simulink model "Test_LQG_non_linear"  (R2022b)
settings: Solver=VariableStepAuto  StartTime=0.0  StopTime=100.0  RelTol=1e-3
values from neighbouring files (symbols this model uses):
  a = Mv+mp+2*ma+2*IAy/(ra^2)    (= 19.1666666667)    [function_f.m]
  b = 1/2*(Mv*l^2+mp*L^2+2*ma*d^2+IGz+IPz+2*IAz+2*IAy*(d/ra)^2)    (= 3.3525)    [function_f.m]
  IPy = 0.15    [function_f.m]
  IPz = 0.23    [function_f.m]
  J = get_linearization()    [DK_iteration.m]    (also in LQG.m; LQG_integrator.m; LQG_with_integrator.m; mu_analysis.m = get_linearization_lqg())
  Kr = lqr(J.A,J.B,Q,R)    [LQG.m]    (also in LQG_integrator.m = lqr(A,B,Q,R); LQG_with_integrator.m = lqr(A,B,Q,R))
  L = 1    [function_f.m]
  rp = 0.3    [function_f.m]
undefined symbols (not defined in the file or in its folder): Ke, std_dev_dx, std_dev_dy, std_dev_phi_dot, std_dev_psi, X_start
libraries: simulink x2
settings Model: Creator=alexi  LastModifiedBy=alexi

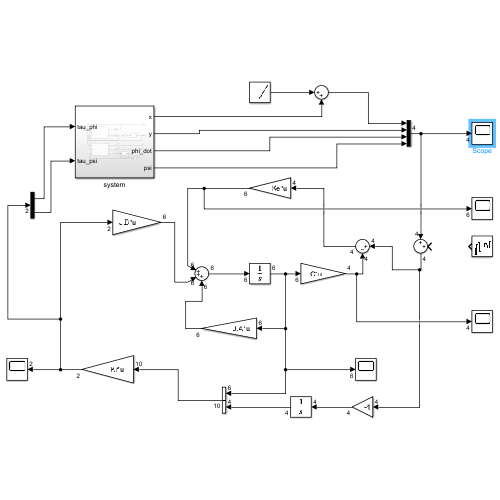
[thumbnail: Simulink's stored preview of the top-level diagram]
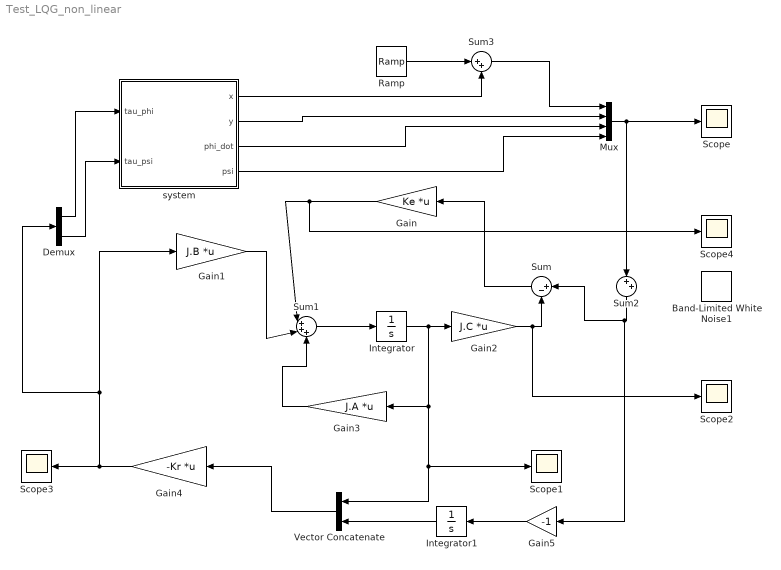
== system Test_LQG_non_linear ==
  Band-Limited White Noise1 : simulink/Sources/Band-Limited White Noise  Cov=[std_dev_dx; std_dev_dy; std_dev_phi_dot; std_dev_psi]  Ts=0.1  seed=[23341]
  Demux : Demux  Outputs=2
  Gain : Gain  Gain=Ke  Multiplication=Matrix(K*u)
  Gain1 : Gain  Gain=J.B  Multiplication=Matrix(K*u)
  Gain2 : Gain  Gain=J.C  Multiplication=Matrix(K*u)
  Gain3 : Gain  Gain=J.A  Multiplication=Matrix(K*u)
  Gain4 : Gain  Gain=-Kr  Multiplication=Matrix(K*u)
  Gain5 : Gain  Gain=-1
  Integrator : Integrator
  Integrator1 : Integrator
  Mux : Mux
  Ramp : simulink/Sources/Ramp  slope=1  start=0  InitialOutput=0
  Scope{,1..4} (5 alike) : Scope
  Sum : Sum  Inputs=|+-
  Sum1 : Sum  Inputs=|+++
  Sum2 : Sum  Inputs=|++
  Sum3 : Sum  Inputs=|++
  Vector Concatenate : Concatenate
  system : Subsystem
  wires:
  Sum1/1 -> Integrator/1
  Gain1/1 -> Sum1/2
  Sum/1 -> Gain/1
  Gain3/1 -> Sum1/3
  Sum2/1 -> Gain5/1, Sum/1
  Integrator/1 -> Vector Concatenate/1, Scope1/1, Gain3/1, Gain2/1
  Gain/1 -> Scope4/1, Sum1/1
  Gain2/1 -> Scope2/1, Sum/2
  Gain4/1 -> Demux/1, Gain1/1, Scope3/1
  Gain5/1 -> Integrator1/1
  Vector Concatenate/1 -> Gain4/1
  Integrator1/1 -> Vector Concatenate/2
  Mux/1 -> Scope/1, Sum2/1
  system/1(x) -> Sum3/2
  Sum3/1 -> Mux/1
  Ramp/1 -> Sum3/1
  system/2(y) -> Mux/2
  system/3(phi_dot) -> Mux/3
  system/4(psi) -> Mux/4
  Demux/1 -> system/1(tau_phi)
  Demux/2 -> system/2(tau_psi)

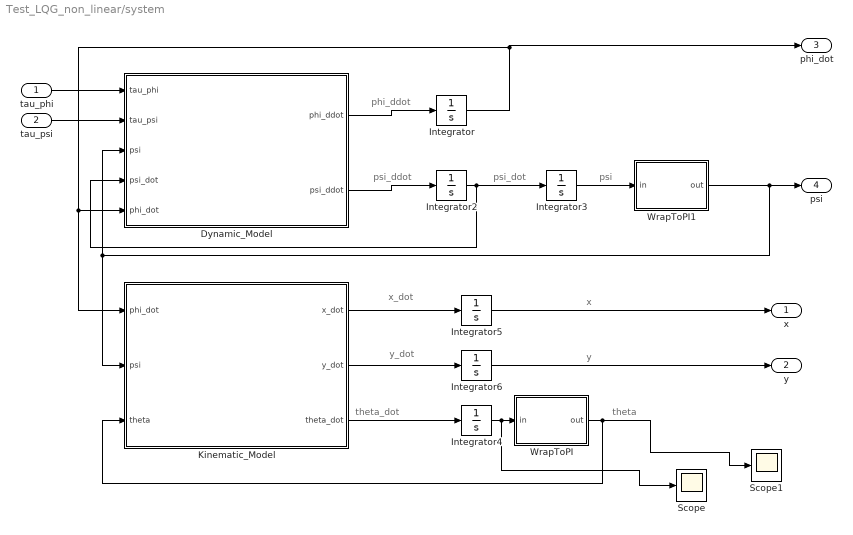
== system Test_LQG_non_linear/system ==
  note: theta_dot
  note: psi_dot
  note: psi_ddot
  note: phi_ddot
  note: psi
  note: theta
  note: x
  note: x_dot
  note: y
  note: y_dot
  tau_phi : Inport
  tau_psi : Inport  Port=2
  Dynamic_Model : MATLAB Function  TreatAsAtomicUnit=on
  Integrator : Integrator  InitialCondition=X_start(4)
  Integrator2 : Integrator  InitialCondition=X_start(6)
  Integrator3 : Integrator  InitialCondition=X_start(5)
  Integrator4 : Integrator  InitialCondition=X_start(3)
  Integrator5 : Integrator  InitialCondition=X_start(1)
  Integrator6 : Integrator  InitialCondition=X_start(2)
  Kinematic_Model : MATLAB Function  TreatAsAtomicUnit=on
  Scope : Scope
  Scope1 : Scope
  WrapToPI : MATLAB Function  TreatAsAtomicUnit=on
  WrapToPI1 : MATLAB Function  TreatAsAtomicUnit=on
  x : Outport
  y : Outport  Port=2
  phi_dot : Outport  Port=3
  psi : Outport  Port=4
  wires:
  Integrator5/1 -> x/1
  Integrator6/1 -> y/1
  WrapToPI1/1(out) -> psi/1, Dynamic_Model/3(psi), Kinematic_Model/2(psi)
  Integrator2/1 -> Integrator3/1, Dynamic_Model/4(psi_dot)
  tau_phi/1 -> Dynamic_Model/1(tau_phi)
  Integrator3/1 -> WrapToPI1/1(in)
  Integrator4/1 -> Scope/1, WrapToPI/1(in)
  Integrator/1 -> Kinematic_Model/1(phi_dot), Dynamic_Model/5(phi_dot), phi_dot/1
  Kinematic_Model/1(x_dot) -> Integrator5/1
  Kinematic_Model/2(y_dot) -> Integrator6/1
  Kinematic_Model/3(theta_dot) -> Integrator4/1
  Dynamic_Model/2(psi_ddot) -> Integrator2/1
  Dynamic_Model/1(phi_ddot) -> Integrator/1
  WrapToPI/1(out) -> Kinematic_Model/3(theta), Scope1/1
  tau_psi/1 -> Dynamic_Model/2(tau_psi)

== matlab function Test_LQG_non_linear/system/Dynamic_Model ==
  data: tau_phi input; tau_psi input; phi_ddot output; psi input; psi_dot input; phi_dot input; psi_ddot output; IPz parameter; IPy parameter; L parameter; rp parameter; b parameter; a parameter
function [phi_ddot,psi_ddot] = DynamicModel(tau_phi,tau_psi,psi,psi_dot,phi_dot,IPz, IPy, L, rp, b, a)
    B = [a*rp^2*cos(psi)^2+b*(rp/L)^2*sin(psi)^2+IPy, -IPz*(rp/L)*sin(psi)
        -IPz*(rp/L)*sin(psi), IPz];
    
    C = [(rp^2*b/L^2-a*rp^2)*cos(psi)*sin(psi)*psi_dot*phi_dot;
            -IPz*rp/L*cos(psi)*psi_dot*phi_dot];

    tau = [tau_phi;
            tau_psi];

    q_ddot = inv(B) * (tau - C);

    phi_ddot = q_ddot(1,:);
    psi_ddot = q_ddot(2,:);

== matlab function Test_LQG_non_linear/system/Kinematic_Model ==
  data: phi_dot input; x_dot output; psi input; theta input; y_dot output; theta_dot output; rp parameter; L parameter
function [x_dot,y_dot,theta_dot] = KinematicModel(phi_dot,psi,theta,rp, L)
    x_dot = rp * phi_dot * cos(theta) * cos(psi);
    y_dot = rp * phi_dot * sin(theta) * cos(psi);
    theta_dot = - (rp * phi_dot * sin(psi)) / L;

== matlab function Test_LQG_non_linear/system/WrapToPI ==
  data: in input; out output
function out = wrapper(in)
    out = wrapTo2Pi(in);

== matlab function Test_LQG_non_linear/system/WrapToPI1 ==
  data: in input; out output
function out = wrapper(in)
    out = wrapToPi(in);
